simulink model "FourLinkSim"  (R2023a)
settings: Solver=ode4  StartTime=0.0  StopTime=1  FixedStep=0.001  RelTol=1e-3
settings Model: Creator=hexia  LastModifiedBy=hexia

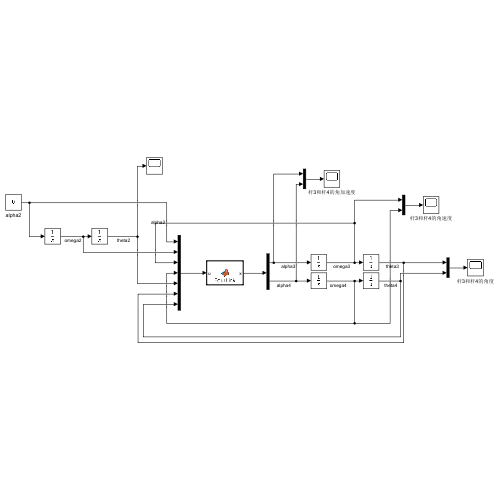
[thumbnail: Simulink's stored preview of the top-level diagram]
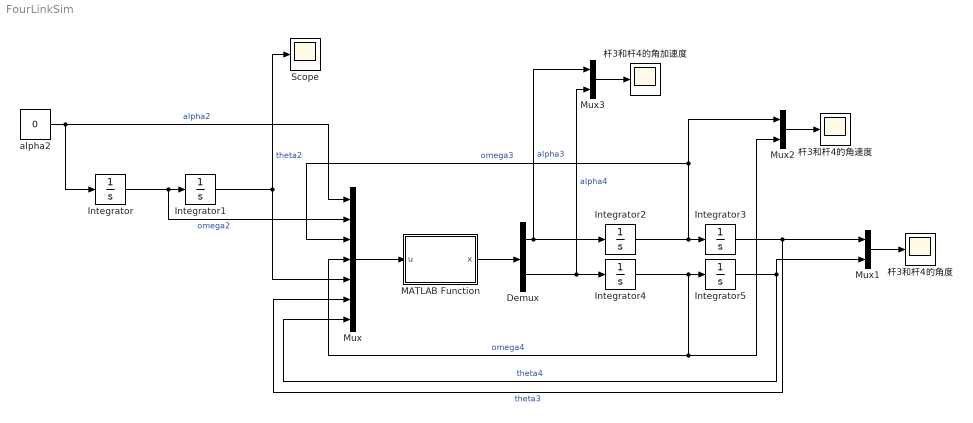
== system FourLinkSim ==
  Demux : Demux  Outputs=2
  Integrator : Integrator  InitialCondition=100
  Integrator1 : Integrator  InitialCondition=45*pi/180
  Integrator2 : Integrator  InitialCondition=-31.319305710416874
  Integrator3 : Integrator  InitialCondition=0.430261050286760
  Integrator4 : Integrator  InitialCondition=21.745437333769640
  Integrator5 : Integrator  InitialCondition=1.582654309064681
  MATLAB Function : MATLAB Function  TreatAsAtomicUnit=on
  Mux : Mux  Inputs=7
  Mux1 : Mux  Inputs=2
  Mux2 : Mux  Inputs=2
  Mux3 : Mux  Inputs=2
  Scope : Scope
  alpha2 : Constant  Value=0
  杆3和杆4的角加速度 : Scope
  杆3和杆4的角度 : Scope
  杆3和杆4的角速度 : Scope
  wires:
  alpha2/1 -> Integrator/1, Mux/1  "alpha2"
  Integrator/1 -> Mux/2, Integrator1/1  "omega2"
  Integrator1/1 -> Scope/1, Mux/5  "theta2"
  Demux/1 -> Mux3/1, Integrator2/1  "alpha3"
  Integrator2/1 -> Mux2/1, Mux/3, Integrator3/1  "omega3"
  Integrator3/1 -> Mux/6, Mux1/1  "theta3"
  Integrator4/1 -> Mux/4, Mux2/2, Integrator5/1  "omega4"
  Demux/2 -> Mux3/2, Integrator4/1  "alpha4"
  Integrator5/1 -> Mux/7, Mux1/2  "theta4"
  MATLAB Function/1(x) -> Demux/1
  Mux/1 -> MATLAB Function/1(u)
  Mux1/1 -> 杆3和杆4的角度/1
  Mux2/1 -> 杆3和杆4的角速度/1
  Mux3/1 -> 杆3和杆4的角加速度/1

== matlab function FourLinkSim/MATLAB Function ==
  data: u input; x output
function x = FourLink(u)
% u(1)=alpha2
% u(2)=omega2
% u(3)=omega3
% u(4)=omega4
% u(5)=theta2
% u(6)=theta3
% u(7)=theta4

% 定义几何尺寸
r1=12.0;
r2=4.0;
r3=10.0;
r4=7.0;

a=[-r3*sin(u(6)) r4*sin(u(7)); r3*cos(u(6)) -r4*cos(u(7))];
b=[r2*u(1)*sin(u(5))+r2*u(2)^2*cos(u(5))+r3*u(3)^2*cos(u(6))-r4*u(4)^2*cos(u(7)); 
   -r2*u(1)*cos(u(5))+r2*u(2)^2*sin(u(5))+r3*u(3)^2*sin(u(6))-r4*u(4)^2*sin(u(7))];
x=inv(a)*b;
